simulink model "h_Controllers"  (R2015a)
settings: Solver=ode2  StartTime=0.0  StopTime=10.0  FixedStep=0.01  RelTol=1e-3
InitFcn:
  | Parameters
values from neighbouring files (symbols this model uses):
  Kdp = 0*0.05    (= 0)    [Parameters.m]
  Kdq = 0*0.05    (= 0)    [Parameters.m]
  Kdr = 0.0001    [Parameters.m]
  Kip = 0*0.3    (= 0)    [Parameters.m]
  Kiq = 0*0.3    (= 0)    [Parameters.m]
  Kir = 0.1    [Parameters.m]
  KPP = 0*1.1    (= 0)    [Parameters.m]
  Kpp = 0*0.3    (= 0)    [Parameters.m]
  Kpq = 0*0.3    (= 0)    [Parameters.m]
  Kpr = 0.05    [Parameters.m]
  KRP = 0*1.1    (= 0)    [Parameters.m]
  KYr = 3    [Parameters.m]
  N = 1/Tf    (= 100)    [Parameters.m]
  pitchMax = pi/6    (= 0.523598775598)    [Parameters.m]
  pitchMin = -pi/6    (= -0.523598775598)    [Parameters.m]
  rollMax = pi/6    (= 0.523598775598)    [Parameters.m]
  rollMin = -pi/6    (= -0.523598775598)    [Parameters.m]
undefined symbols (not defined in the file or in its folder): KPD, KRD
libraries: simulink x5
settings Model: Creator=pela  LastModifiedBy=pela
settings HardwareCC: ProdLargestAtomicInteger=Long  ProdLargestAtomicFloat=Double  ProdEndianess=LittleEndian  ProdHWDeviceType=ARM Compatible->ARM Cortex
settings RTWCC: GenCodeOnly=on  GenerateReport=on  BuildConfiguration=Faster Runs  LaunchReport=on  TargetLang=C++
settings GRTTargetCC: MatFileLogging=off  MultiInstanceERTCode=on  CodeInterfacePackaging=C++ class  SupportNonFinite=off

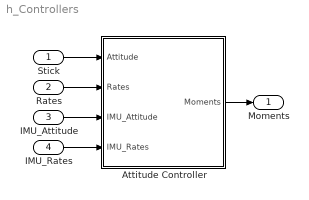
== system h_Controllers ==
  Stick : Inport
  Rates : Inport  Port=2
  IMU_Attitude : Inport  Port=3
  IMU_Rates : Inport  Port=4
  Attitude Controller : Subsystem
  Moments : Outport
  wires:
  Attitude Controller/1(Moments) -> Moments/1
  Stick/1 -> Attitude Controller/1(Attitude)
  IMU_Attitude/1 -> Attitude Controller/3(IMU_Attitude)
  IMU_Rates/1 -> Attitude Controller/4(IMU_Rates)
  Rates/1 -> Attitude Controller/2(Rates)

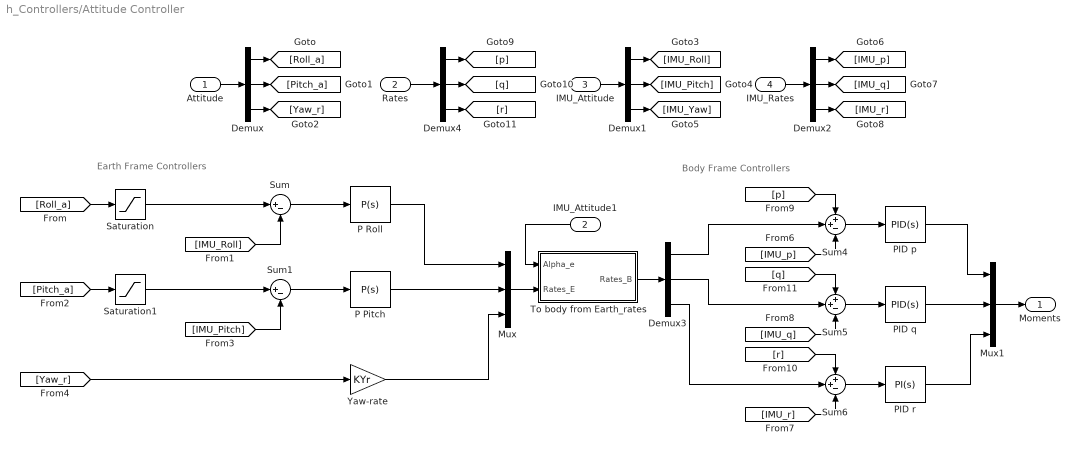
== system h_Controllers/Attitude Controller ==
  note: Body Frame Controllers
  note: Earth Frame Controllers
  Attitude : Inport
  Rates : Inport  Port=2
  IMU_Attitude : Inport  Port=3
  IMU_Rates : Inport  Port=4
  Demux{,1..4} (5 alike) : Demux  Outputs=3
  IMU_Attitude1 : InportShadow  Port=2
  Mux : Mux  Inputs=3
  Mux1 : Mux  Inputs=3
  P Pitch : simulink/Continuous/PID Controller  Controller=P  TimeDomain=Continuous-time  SampleTime=-1  IntegratorMethod=Forward Euler  FilterMethod=Forward Euler  Form=Parallel  UseFilter=on  ControllerParametersSource=internal  P=KPP  I=Kip  D=KPD  N=N  InitialConditionSource=internal  InitialConditionForIntegrator=0  InitialConditionForFilter=0  ExternalReset=none  LimitOutput=off  UpperSaturationLimit=inf  LowerSaturationLimit=-inf  LinearizeAsGain=on  AntiWindupMode=none  Kb=1  TrackingMode=off  Kt=1  PParamMin=[]  PParamMax=[]  IParamMin=[]  IParamMax=[]  DParamMin=[]  DParamMax=[]  NParamMin=[]  NParamMax=[]  KbParamMin=[]  KbParamMax=[]  KtParamMin=[]  KtParamMax=[]  POutMin=[]  POutMax=[]  IOutMin=[]  IOutMax=[]  DOutMin=[]  DOutMax=[]  NOutMin=[]  NOutMax=[]  KbOutMin=[]  KbOutMax=[]  KtOutMin=[]  KtOutMax=[]  IntegratorOutMin=[]  IntegratorOutMax=[]  FilterOutMin=[]  FilterOutMax=[]  SumOutMin=[]  SumOutMax=[]  SumI1OutMin=[]  SumI1OutMax=[]  SumI2OutMin=[]  SumI2OutMax=[]  SumI3OutMin=[]  SumI3OutMax=[]  SumDOutMin=[]  SumDOutMax=[]  SaturationOutMin=[]  SaturationOutMax=[]  IntegratorContinuousStateAttributes=''  IntegratorStateMustResolveToSignalObject=off  IntegratorRTWStateStorageClass=Auto  FilterContinuousStateAttributes=''  FilterStateMustResolveToSignalObject=off  FilterRTWStateStorageClass=Auto  DifferentiatorICPrevScaledInput=0  DifferentiatorOutMin=[]  DifferentiatorOutMax=[]
  P Roll : simulink/Continuous/PID Controller  Controller=P  TimeDomain=Continuous-time  SampleTime=-1  IntegratorMethod=Forward Euler  FilterMethod=Forward Euler  Form=Parallel  UseFilter=on  ControllerParametersSource=internal  P=KRP  I=Kip  D=KRD  N=N  InitialConditionSource=internal  InitialConditionForIntegrator=0  InitialConditionForFilter=0  ExternalReset=none  LimitOutput=off  UpperSaturationLimit=inf  LowerSaturationLimit=-inf  LinearizeAsGain=on  AntiWindupMode=none  Kb=1  TrackingMode=off  Kt=1  PParamMin=[]  PParamMax=[]  IParamMin=[]  IParamMax=[]  DParamMin=[]  DParamMax=[]  NParamMin=[]  NParamMax=[]  KbParamMin=[]  KbParamMax=[]  KtParamMin=[]  KtParamMax=[]  POutMin=[]  POutMax=[]  IOutMin=[]  IOutMax=[]  DOutMin=[]  DOutMax=[]  NOutMin=[]  NOutMax=[]  KbOutMin=[]  KbOutMax=[]  KtOutMin=[]  KtOutMax=[]  IntegratorOutMin=[]  IntegratorOutMax=[]  FilterOutMin=[]  FilterOutMax=[]  SumOutMin=[]  SumOutMax=[]  SumI1OutMin=[]  SumI1OutMax=[]  SumI2OutMin=[]  SumI2OutMax=[]  SumI3OutMin=[]  SumI3OutMax=[]  SumDOutMin=[]  SumDOutMax=[]  SaturationOutMin=[]  SaturationOutMax=[]  IntegratorContinuousStateAttributes=''  IntegratorStateMustResolveToSignalObject=off  IntegratorRTWStateStorageClass=Auto  FilterContinuousStateAttributes=''  FilterStateMustResolveToSignalObject=off  FilterRTWStateStorageClass=Auto  DifferentiatorICPrevScaledInput=0  DifferentiatorOutMin=[]  DifferentiatorOutMax=[]
  PID p : simulink/Continuous/PID Controller  Controller=PID  TimeDomain=Continuous-time  SampleTime=-1  IntegratorMethod=Forward Euler  FilterMethod=Forward Euler  Form=Parallel  UseFilter=on  ControllerParametersSource=internal  P=Kpp  I=Kip  D=Kdp  N=N  InitialConditionSource=internal  InitialConditionForIntegrator=0  InitialConditionForFilter=0  ExternalReset=none  LimitOutput=off  UpperSaturationLimit=inf  LowerSaturationLimit=-inf  LinearizeAsGain=on  AntiWindupMode=none  Kb=1  TrackingMode=off  Kt=1  PParamMin=[]  PParamMax=[]  IParamMin=[]  IParamMax=[]  DParamMin=[]  DParamMax=[]  NParamMin=[]  NParamMax=[]  KbParamMin=[]  KbParamMax=[]  KtParamMin=[]  KtParamMax=[]  POutMin=[]  POutMax=[]  IOutMin=[]  IOutMax=[]  DOutMin=[]  DOutMax=[]  NOutMin=[]  NOutMax=[]  KbOutMin=[]  KbOutMax=[]  KtOutMin=[]  KtOutMax=[]  IntegratorOutMin=[]  IntegratorOutMax=[]  FilterOutMin=[]  FilterOutMax=[]  SumOutMin=[]  SumOutMax=[]  SumI1OutMin=[]  SumI1OutMax=[]  SumI2OutMin=[]  SumI2OutMax=[]  SumI3OutMin=[]  SumI3OutMax=[]  SumDOutMin=[]  SumDOutMax=[]  SaturationOutMin=[]  SaturationOutMax=[]  IntegratorContinuousStateAttributes=''  IntegratorStateMustResolveToSignalObject=off  IntegratorRTWStateStorageClass=Auto  FilterContinuousStateAttributes=''  FilterStateMustResolveToSignalObject=off  FilterRTWStateStorageClass=Auto  DifferentiatorICPrevScaledInput=0  DifferentiatorOutMin=[]  DifferentiatorOutMax=[]
  PID q : simulink/Continuous/PID Controller  Controller=PID  TimeDomain=Continuous-time  SampleTime=-1  IntegratorMethod=Forward Euler  FilterMethod=Forward Euler  Form=Parallel  UseFilter=on  ControllerParametersSource=internal  P=Kpq  I=Kiq  D=Kdq  N=N  InitialConditionSource=internal  InitialConditionForIntegrator=0  InitialConditionForFilter=0  ExternalReset=none  LimitOutput=off  UpperSaturationLimit=inf  LowerSaturationLimit=-inf  LinearizeAsGain=on  AntiWindupMode=none  Kb=1  TrackingMode=off  Kt=1  PParamMin=[]  PParamMax=[]  IParamMin=[]  IParamMax=[]  DParamMin=[]  DParamMax=[]  NParamMin=[]  NParamMax=[]  KbParamMin=[]  KbParamMax=[]  KtParamMin=[]  KtParamMax=[]  POutMin=[]  POutMax=[]  IOutMin=[]  IOutMax=[]  DOutMin=[]  DOutMax=[]  NOutMin=[]  NOutMax=[]  KbOutMin=[]  KbOutMax=[]  KtOutMin=[]  KtOutMax=[]  IntegratorOutMin=[]  IntegratorOutMax=[]  FilterOutMin=[]  FilterOutMax=[]  SumOutMin=[]  SumOutMax=[]  SumI1OutMin=[]  SumI1OutMax=[]  SumI2OutMin=[]  SumI2OutMax=[]  SumI3OutMin=[]  SumI3OutMax=[]  SumDOutMin=[]  SumDOutMax=[]  SaturationOutMin=[]  SaturationOutMax=[]  IntegratorContinuousStateAttributes=''  IntegratorStateMustResolveToSignalObject=off  IntegratorRTWStateStorageClass=Auto  FilterContinuousStateAttributes=''  FilterStateMustResolveToSignalObject=off  FilterRTWStateStorageClass=Auto  DifferentiatorICPrevScaledInput=0  DifferentiatorOutMin=[]  DifferentiatorOutMax=[]
  PID r : simulink/Continuous/PID Controller  Controller=PI  TimeDomain=Continuous-time  SampleTime=-1  IntegratorMethod=Forward Euler  FilterMethod=Forward Euler  Form=Parallel  UseFilter=on  ControllerParametersSource=internal  P=Kpr  I=Kir  D=Kdr  N=N  InitialConditionSource=internal  InitialConditionForIntegrator=0  InitialConditionForFilter=0  ExternalReset=none  LimitOutput=off  UpperSaturationLimit=inf  LowerSaturationLimit=-inf  LinearizeAsGain=on  AntiWindupMode=none  Kb=1  TrackingMode=off  Kt=1  PParamMin=[]  PParamMax=[]  IParamMin=[]  IParamMax=[]  DParamMin=[]  DParamMax=[]  NParamMin=[]  NParamMax=[]  KbParamMin=[]  KbParamMax=[]  KtParamMin=[]  KtParamMax=[]  POutMin=[]  POutMax=[]  IOutMin=[]  IOutMax=[]  DOutMin=[]  DOutMax=[]  NOutMin=[]  NOutMax=[]  KbOutMin=[]  KbOutMax=[]  KtOutMin=[]  KtOutMax=[]  IntegratorOutMin=[]  IntegratorOutMax=[]  FilterOutMin=[]  FilterOutMax=[]  SumOutMin=[]  SumOutMax=[]  SumI1OutMin=[]  SumI1OutMax=[]  SumI2OutMin=[]  SumI2OutMax=[]  SumI3OutMin=[]  SumI3OutMax=[]  SumDOutMin=[]  SumDOutMax=[]  SaturationOutMin=[]  SaturationOutMax=[]  IntegratorContinuousStateAttributes=''  IntegratorStateMustResolveToSignalObject=off  IntegratorRTWStateStorageClass=Auto  FilterContinuousStateAttributes=''  FilterStateMustResolveToSignalObject=off  FilterRTWStateStorageClass=Auto  DifferentiatorICPrevScaledInput=0  DifferentiatorOutMin=[]  DifferentiatorOutMax=[]
  Saturation : Saturate  UpperLimit=rollMax  LowerLimit=rollMin
  Saturation1 : Saturate  UpperLimit=pitchMax  LowerLimit=pitchMin
  Sum : Sum  Inputs=|+-
  Sum1 : Sum  Inputs=|+-
  Sum4 : Sum  Inputs=++-
  Sum5 : Sum  Inputs=++-
  Sum6 : Sum  Inputs=++-
  To body from Earth_rates : MATLAB Function  TreatAsAtomicUnit=on
  Yaw-rate : Gain  Gain=KYr
  Moments : Outport
  wires:
  Yaw-rate/1 -> Mux/3
  Sum4/1 -> PID p/1
  IMU_Attitude/1 -> Demux1/1
  Attitude/1 -> Demux/1
  Demux/3 -> [Yaw_r]
  IMU_Rates/1 -> Demux2/1
  [IMU_Pitch] -> Sum1/2
  [Pitch_a] -> Saturation1/1
  [IMU_Roll] -> Sum/2
  [Roll_a] -> Saturation/1
  Mux1/1 -> Moments/1
  P Roll/1 -> Mux/1
  [Yaw_r] -> Yaw-rate/1
  P Pitch/1 -> Mux/2
  [IMU_r] -> Sum6/3
  Sum5/1 -> PID q/1
  PID r/1 -> Mux1/3
  PID p/1 -> Mux1/1
  Sum6/1 -> PID r/1
  PID q/1 -> Mux1/2
  Demux/2 -> [Pitch_a]
  Demux2/3 -> [IMU_r]
  Demux1/1 -> [IMU_Roll]
  Demux/1 -> [Roll_a]
  Demux2/1 -> [IMU_p]
  Demux1/3 -> [IMU_Yaw]
  Demux2/2 -> [IMU_q]
  Demux1/2 -> [IMU_Pitch]
  Sum/1 -> P Roll/1
  Sum1/1 -> P Pitch/1
  Saturation/1 -> Sum/1
  Saturation1/1 -> Sum1/1
  Demux3/1 -> Sum4/2
  [p] -> Sum4/1
  [IMU_p] -> Sum4/3
  Rates/1 -> Demux4/1
  Demux4/3 -> [r]
  Demux4/2 -> [q]
  Demux4/1 -> [p]
  [q] -> Sum5/1
  [IMU_q] -> Sum5/3
  [r] -> Sum6/1
  Demux3/2 -> Sum5/2
  Demux3/3 -> Sum6/2
  IMU_Attitude1/1 -> To body from Earth_rates/1(Alpha_e)
  To body from Earth_rates/1(Rates_B) -> Demux3/1
  Mux/1 -> To body from Earth_rates/2(Rates_E)

== matlab function h_Controllers/Attitude Controller/To body from Earth_rates ==
  data: Alpha_e input; Rates_B output; Rates_E input
 function Rates_B = E(Alpha_e, Rates_E)
%#codegen
phi = Alpha_e(1);
theta = Alpha_e(2);

Sphi = sin(phi);
Cphi = cos(phi);
Stheta = sin(theta);
Ctheta = cos(theta);

E = [1      0        -Stheta   ;
     0     Cphi    Sphi*Ctheta ;
     0    -Sphi    Cphi*Ctheta];

Rates_B = E* Rates_E;
